simulink model "43_BusNetworkElectricityTransmissionModel"  (R2023b)
settings: Solver=VariableStepAuto  StartTime=0.0  StopTime=0.8  RelTol=1e-3
model workspace (MAT data in the model file):
  BESS_Fp_KDroop = 0.025
  BESS_KSI = 817
  BESS_PWM_fs = 560
  BESS_P_Ki = 0.5
  BESS_P_Kp = 0.0636
  BESS_Pnom = 3000000
  BESS_Q_Ki = 1
  BESS_Q_Kp = 0.0257
  BESS_Vd_Ki = 850
  BESS_Vd_Kp = 0.216
  BESS_Vnom = 1000
  BESS_Vq_KDroop = 0.025
  BESS_Vq_Ki = 850
  BESS_Vq_Kp = 0.216
  Compensation_Ki = 30
  Compensation_Kp = 3
  DC_Ki = 400
  DC_Kp = 8
  F = 0.01
  Flux_min = 0.5
  Grid_Freq_PWM = 2700
  Grid_Ireg_Ki = 5
  Grid_Ireg_Kp = 0.83
  Grid_Ireg_lim = 1.1
  Grid_Modindex_Upper = 1.1
  Grid_conv_Imax = 0.8
  H = 0.685
  Idref_max = 0.9
  Iqref_Tc = 0.3
  Ki_Var = 0.05
  Ki_Vreg = 20
  Ksh = 1.1
  L_pu = 0.3
  Llr = 0.16
  Lls = 0.18
  Lm = 2.9
  LowLoad_P = 130
  Nb_wt = 6
  P_mech = 1080000
  PeakShav_P = 200
  Pitch_Ki = 0
  Pitch_Kp = 150
  Pitch_Max = 27
  Pitch_Tc = 0.01
  Pitch_rate = 10
  Q_Filt = 50
  R_pu = 0.003
  Rotor_Freq_PWM = 1620
  Rotor_Ireg_Ki = 8
  Rotor_Ireg_Kp = 0.6
  Rotor_Ireg_lim = 0.1
  Rotor_Modindex_Upper = 2
  Rr = 0.016
  Rs = 0.023
  SOCBESS = Simulink.Parameter
  SOCBESS.DataType = 'auto'
  SOCBESS.Complexity = 'real'
  SOCBESS.Dimensions = [0 0]
  T_set = 0.0001
  Tp = 5e-05
  Ts = 5e-06
  Var_C_Filt = 720000
  Var_reg_max = 1.1
  Var_reg_min = 0.9
  WT_Coeff = [0.645 116 0.4 5 21 0.00912 0.08 0.035]
  WT_H = 4.32
  WT_IGBTRon = 5.931
  WT_Param = [91.204 10143]
  Wind_Freq_Filt = 10000
  Wind_Freq_nom = 60
  Wind_P_nom = 1200000
  Wind_Rotor_V_nom = 1950
  Wind_V_nom = 500
  Zeta_Filt = 0.707106781187
  init = [-0.2 0 0 0 0 0 0 0]
  p = 3
  torque0 = 0.83
  v_Ki = 0.1
  v_Kp = 3.6
  v_Max = 1.2
  v_Min = 0.7
  v_T = 5
  vreg_max = 1
  wind_VDC_nom = 1150
  wt0 = 1.2
undefined symbols (not defined in the file): D1, D11, Delta, DiscIntNeverNeededParam, Iabc, Ion, Lithium, P, Q, Vabc
libraries: powerlib_extras x156, spsSeriesRLCBranchLib x66, spsLoadFlowBusLib x43, spsThreePhaseSeriesRLCLoadLib x33, spsThreePhaseTransformerTwoWindingsLib x32, spsThreePhaseVIMeasurementLib x30, simulink_extras x30, spsDistributedParametersLineLib x22, spsGenericPowerSystemStabilizerLib x20, spsSynchronousMachinepuStandardLib x10, spsExcitationSystemLib x10, spsHydraulicTurbineandGovernorLib x10
(part 1 of 19)
settings Model: Creator=3.22  LastModifiedBy=3.22

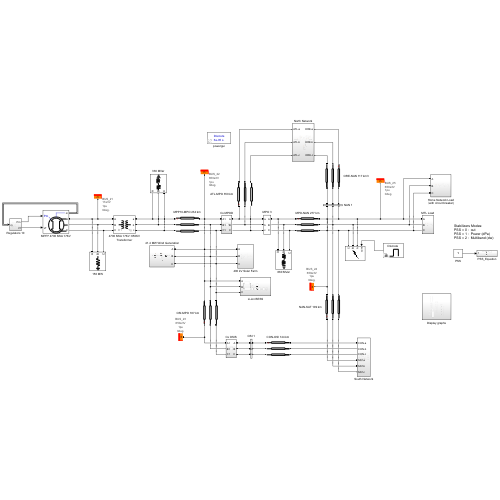
[thumbnail: Simulink's stored preview of the top-level diagram]
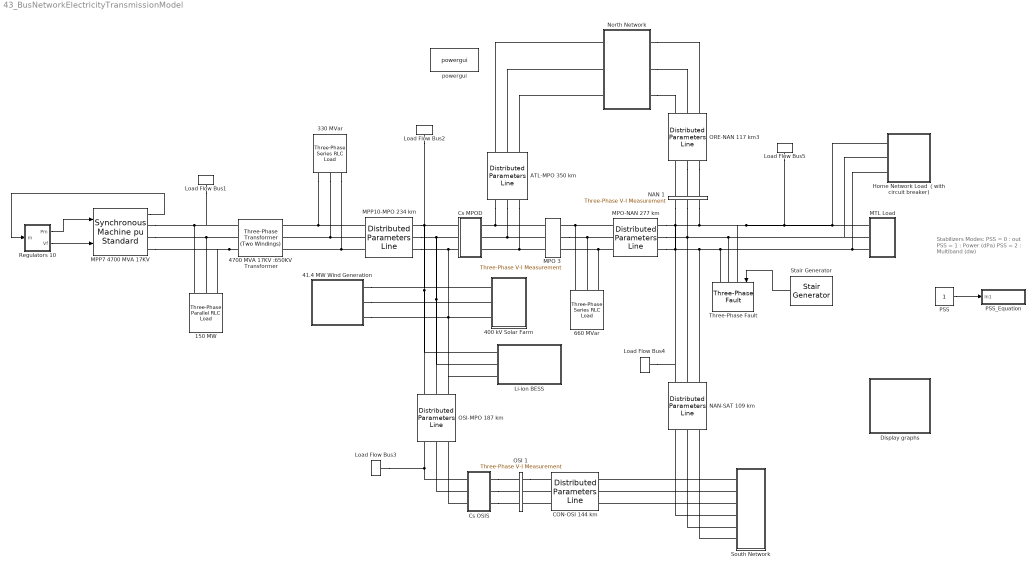
== system 43_BusNetworkElectricityTransmissionModel ==
  note: Stabilizers Modes:
      | PSS = 0 :  out
      | PSS = 1 :  Power (dPa)
      | PSS = 2 :  Multiband (dw)
  " 41.4 MW Wind Generation" : Subsystem
  150 MW : spsThreePhaseParallelRLCLoadLib/Three-Phase Parallel RLC Load  LConnTagsString=A|B|C  Configuration=Y (grounded)  NominalVoltage=17000  Vabc=[1e3 1e3 1e3]  Vabcp=[1e3 1e3 1e3]  NominalFrequency=60  UnbalancedPower=off  ActivePower=150e6  InductivePower=0  CapacitivePower=0  Pabc=[10e3 9e3 11e3]  QLabc=[100 90 110]  QCabc=[100 90 110]  Pabcp=[10e3 9e3 11e3]  QLabcp=[100 90 110]  QCabcp=[100 90 110]  Measurements=None  LoadType=constant Z
  330 MVar : spsThreePhaseSeriesRLCLoadLib/Three-Phase Series RLC Load  LConnTagsString=A|B|C  Configuration=Y (grounded)  NominalVoltage=650e3  Vabc=[1e3 1e3 1e3]  Vabcp=[1e3 1e3 1e3]  NominalFrequency=60  UnbalancedPower=off  ActivePower=1100e3  InductivePower=330e6  CapacitivePower=0  Pabc=[10e3 9e3 11e3]  QLabc=[100 90 110]  QCabc=[100 90 110]  Pabcp=[10e3 9e3 11e3]  QLabcp=[100 90 110]  QCabcp=[100 90 110]  Measurements=None  LoadType=constant Z
  400 kV Solar Farm : Subsystem
  "4700 MVA 17KV :650KV Transformer " : spsThreePhaseTransformerTwoWindingsLib/Three-Phase Transformer (Two Windings)  Winding1Connection=Delta (D1)  Winding2Connection=Yg  CoreType=Three single-phase transformers  SetSaturation=off  Hysteresis=off  DataFile='hysteresis'  SetInitialFlux=off  Measurements=None  UNITS=pu  NominalPower=[ 4700e6 , 60 ]  Winding1=[ 17e3 , 0.002 , 0.08 ]  Winding2=[ 650e3 , 0.002 , 0.08 ]  Rm=500  Lm=500  L0=0.5  Saturation=[ 0,0 ; 0.0024,1.2 ; 1.0,1.52 ]  InitialFluxes=[ 0.8 , -0.8 , 0.7 ]  BreakLoop=off  DiscreteSolver=Trapezoidal iterative  DataType=off  TransfoNumber=1
  660 MVar : spsThreePhaseSeriesRLCLoadLib/Three-Phase Series RLC Load  LConnTagsString=A|B|C  Configuration=Y (grounded)  NominalVoltage=650e3  Vabc=[1e3 1e3 1e3]  Vabcp=[1e3 1e3 1e3]  NominalFrequency=60  UnbalancedPower=off  ActivePower=2200e3  InductivePower=660e6  CapacitivePower=0  Pabc=[10e3 9e3 11e3]  QLabc=[100 90 110]  QCabc=[100 90 110]  Pabcp=[10e3 9e3 11e3]  QLabcp=[100 90 110]  QCabcp=[100 90 110]  Measurements=None  LoadType=constant Z
  ATL-MPO 350 km : spsDistributedParametersLineLib/Distributed Parameters Line  Phases=3  Length=350  Frequency=60  Resistance=[0.01273 0.3864]/6  Inductance="[0.9337e-3  4.1264e-3]/6"  Capacitance=[12.74e-9 7.751e-9]*6  x1=[-0.00198 6.71985344224008e-09 -287571.845218076 -158091.891979352;-0.00192 6.70807661913084e-09 -283922.60888035 -164555.645992495;-0.00186 6.69286782007226e-09 -280128.112489635 -170935.210296509;-0.0018 6.67423482616695e-09 -276190.297380398 -177227.320988416;-0.00174 6.65218717039889e-09 -272111.17821161 -183428.758908121;-0.00168 6.62673613275617e-09 -267892.841936014 -189536.351285395;-0.00162 6.59789473445993e-09 -263537.446732392 -195546.973363122;-0.00156 6.56567773130246e-09 -259047.22090141 -201457.549995984;-0.0015 6.53010160609788e-09 -254424.461725573 -207265.05722376;-0.00144 6.49118456024921e-09 -249671.534293893 -212966.523818443;-0.00138 6.44894650443622e-09 -244790.870291869 -218559.032804371;-0.00132 6.40340904842874e-09 -239784.966757388 -224039.722950611;-0.00126 6.35459549003068e-09 -234656.384803197 -229405.79023481;-0.0012 6.30253080316049e-09 -229407.74830659 -234654.489277794;-0.00114 6.24724162507404e-09 -224041.742566981 -239783.134748147;-0.00108 6.18875624273644e-09 -218561.11293206 -244789.102736079;-0.00102 6.12710457834999e-09 -212968.663393218 -249669.83209587;-0.00096 6.06231817404538e-09 -207267.255150975 -254422.825756192;-0.0009 5.99443017574417e-09 -201459.805151138 -259045.651997664;-0.00084 5.92347531620071e-09 -195549.284592437 -263535.94569696;-0.00078 5.84948989723225e-09 -189538.717406403 -267891.409536854;-0.00072 5.77251177114621e-09 -183431.178710271 -272109.815181565;-0.00066 5.69258032137431e-09 -177229.793233693 -276189.004416817;-0.0006 5.6097364423232e-09 -170937.733720066 -280126.890254024;-0.00054 5.52402251845218e-09 -164558.219303301 -283921.457998027;-0.00048 5.43548240258853e-09 -158094.513860855 -287570.766277852;-0.00042 5.34416139349154e-09 -151549.924343867 -291072.948039954;-0.00036 5.25010621267689e-09 -144927.799085264 -294426.211503428;-0.0003 5.15336498051303e-09 -138231.526086691 -297628.841076726;-0.00024 5.05398719160191e-09 -131464.531285147 -300679.198235381;-0.00018 4.95202368945661e-09 -124630.276800213 -303575.722360306;-0.00012 4.84752664048891e-09 -117732.259162765 -306316.931536237;-6e-05 4.74054950731994e-09 -110774.007526087 -308901.423309907]  x2=[-0.00198 2.79653655239106e-09 -267672.30015696 -181652.17479948;-0.00192 2.55125047403786e-09 -263495.280738514 -187659.824526183;-0.00186 2.30465912880045e-09 -259183.45226561 -193571.464019103;-0.0018 2.05688867736754e-09 -254739.020749366 -199384.068774241;-0.00174 1.80806588368036e-09 -250164.260043072 -205094.664955601;-0.00168 1.55831805007787e-09 -245461.510678835 -210700.330916655;-0.00162 1.30777295216655e-09 -240633.178670128 -216198.198695118;-0.00156 1.05655877344804e-09 -235681.734280824 -221585.455480246;-0.0015 8.04804039738072e-10 -230609.710761363 -226859.345051921;-0.00144 5.52637553410303e-10 -225419.7030527 -232017.169190789;-0.00138 3.00188327498644e-10 -220114.366458677 -237056.289058714;-0.00132 4.75855196917935e-11 -214696.415287529 -241974.126548861;-0.00126 -2.05041633746211e-10 -209168.621463186 -246768.165604697;-0.0012 -4.57563884095656e-10 -203533.81310711 -251435.953507259;-0.00114 -7.0985203630719e-10 -197794.873091376 -255975.102130004;-0.00108 -9.61777015100393e-10 -191954.73756374 -260383.289160623;-0.00102 -1.21320993100107e-09 -186016.394445451 -264658.259289177;-0.00096 -1.46402214628351e-09 -179982.881902575 -268797.825361957;-0.0009 -1.71408534078389e-09 -173857.286791617 -272799.869500469;-0.00084 -1.96327157755127e-09 -167642.743080223 -276662.344184983;-0.00078 -2.21145336830249e-09 -161342.430243787 -280383.273302079;-0.00072 -2.45850373864752e-09 -154959.571638773 -283960.753155667;-0.00066 -2.70429629305194e-09 -148497.432853586 -287392.953440949;-0.0006 -2.94870527950318e-09 -141959.320037833 -290678.118180839;-0.00054 -3.19160565384762e-09 -135348.578210842 -293814.566624354;-0.00048 -3.43287314376546e-09 -128668.589550285 -296800.694106514;-0.00042 -3.67238431235074e-09 -121922.771661791 -299634.972869324;-0.00036 -3.91001662126397e-09 -115114.575830441 -302315.952843396;-0.0003 -4.14564849342495e-09 -108247.485255024 -304842.262389837;-0.00024 -4.37915937521393e-09 -101325.013265967 -307212.609002002;-0.00018 -4.61042979814898e-09 -94350.7015278514 -309425.779966765;-0.00012 -4.83934144000835e-09 -87328.118227434 -311480.642984966;-6e-05 -5.06577718536627e-09 -80260.8562480934 -313376.146750715]  x3=[-0.00198 1.49045766658214e-10 -8241.07227031755 -3031.05749753974;-0.00192 1.47930956165664e-10 -8170.40834869366 -3216.6754938586;-0.00186 1.46740461462489e-10 -8095.56429518679 -3400.64777955748;-0.0018 1.45474891627779e-10 -8016.57840139768 -3582.88023101559;-0.00174 1.44134894150444e-10 -7933.49107796907 -3763.27961474349;-0.00168 1.42721154597956e-10 -7846.34483391092 -3941.75363508309;-0.00162 1.41234396265592e-10 -7755.18425485195 -4118.21098142774;-0.00156 1.39675379806387e-10 -7660.05598022887 -4292.5613749385;-0.0015 1.38044902841968e-10 -7561.00867942474 -4464.71561473243;-0.00144 1.36343799554479e-10 -7458.09302686885 -4634.5856235194;-0.00138 1.34572940259794e-10 -7351.36167611069 -4802.08449266409;-0.00132 1.3273323096225e-10 -7240.86923288149 -4967.12652665;-0.00126 1.30825612891118e-10 -7126.67222715687 -5129.62728692295;-0.0012 1.28851062019051e-10 -7008.82908423508 -5289.50363509128;-0.00114 1.26810588562762e-10 -6887.40009484551 -5446.67377546111;-0.00108 1.24705236466173e-10 -6762.44738430291 -5601.05729688446;-0.00102 1.22536082866321e-10 -6634.03488072283 -5752.57521389908;-0.00096 1.20304237542268e-10 -6502.22828231491 -5901.15000713891;-0.0009 1.18010842347321e-10 -6367.09502377039 -6046.70566299436;-0.00084 1.1565707062484e-10 -6228.70424176131 -6189.16771250235;-0.00078 1.1324412660793e-10 -6087.12673956894 -6328.46326944596;-0.00072 1.10773244803337e-10 -5942.43495085943 -6464.52106764436;-0.00066 1.08245689359848e-10 -5794.70290262548 -6597.27149741394;-0.0006 1.05662753421532e-10 -5644.00617731276 -6726.64664118189;-0.00054 1.03025758466143e-10 -5490.42187415047 -6852.58030823406;-0.00048 1.00336053629025e-10 -5334.02856970605 -6975.00806857942;-0.00042 9.75950150128734e-11 -5174.90627768384 -7093.86728591356;-0.00036 9.48040449836927e-11 -5013.1364079887 -7209.09714966463;-0.0003 9.19645714533211e-11 -4848.80172507512 -7320.63870610513;-0.00024 8.9078047148884e-11 -4681.98630560344 -7428.43488851374;-0.00018 8.61459488695525e-11 -4512.77549542465 -7532.4305463717;-0.00012 8.31697767309852e-11 -4341.25586591589 -7632.57247357881;-6e-05 8.01510533978416e-11 -4167.51516968895 -7728.80943567472]  x4=[-0.00198 -4.77653400589125e-11 -5640.6008243666 -1578.68999483631;-0.00192 -4.78138362701717e-11 -5603.45127275738 -1705.86309036725;-0.00186 -4.78378700392969e-11 -5563.43489193714 -1832.16343482044;-0.0018 -4.78374290701678e-11 -5520.57215502573 -1957.52641060589;-0.00174 -4.78125135883924e-11 -5474.88499139136 -2081.88787970874;-0.00168 -4.77631363411914e-11 -5426.39677543116 -2205.18421650347;-0.00162 -4.76893225908771e-11 -5375.13231461236 -2327.35234030591;-0.00156 -4.75911101019278e-11 -5321.11783678037 -2448.32974764653;-0.0015 -4.74685491216678e-11 -5264.38097674014 -2568.05454424832;-0.00144 -4.73217023545593e-11 -5204.95076211764 -2686.46547669308;-0.00138 -4.71506449301216e-11 -5142.8575985088 -2803.50196375979;-0.00132 -4.69554643644939e-11 -5078.13325392348 -2919.10412741908;-0.00126 -4.67362605156601e-11 -5010.81084253234 -3033.21282346794;-0.0012 -4.64931455323597e-11 -4940.92480772502 -3145.76967178898;-0.00114 -4.62262437967104e-11 -4868.51090448828 -3256.7170862188;-0.00108 -4.59356918605719e-11 -4793.60618111307 -3365.9983040101;-0.00102 -4.56216383756836e-11 -4716.24896023993 -3473.55741487256;-0.00096 -4.52842440176113e-11 -4636.47881925248 -3579.33938957762;-0.0009 -4.4923681403543e-11 -4554.33657002882 -3683.29010811238;-0.00084 -4.45401350039744e-11 -4469.86423806147 -3785.35638736845;-0.00078 -4.41338010483308e-11 -4383.10504095633 -3885.4860083514;-0.00072 -4.37048874245719e-11 -4294.10336632177 -3983.62774289696;-0.00066 -4.32536135728331e-11 -4202.9047490591 -4079.73137988027;-0.0006 -4.27802103731556e-11 -4109.55584806605 -4173.74775090486;-0.00054 -4.22849200273638e-11 -4014.10442236527 -4265.6287554581;-0.00048 -4.17679959351505e-11 -3916.59930666989 -4355.3273855203;-0.00042 -4.1229702564433e-11 -3817.09038639878 -4442.79774961486;-0.00036 -4.06703153160462e-11 -3715.62857215427 -4527.99509628725;-0.0003 -4.00901203828427e-11 -3612.26577367532 -4610.87583700066;-0.00024 -3.9489414603271e-11 -3507.05487327957 -4691.39756843667;-0.00018 -3.88685053095079e-11 -3400.04969880772 -4769.5190941896;-0.00012 -3.8227710170221e-11 -3291.30499608426 -4845.20044584337;-6e-05 -3.75673570280441e-11 -3180.87640090849 -4918.40290342003]  x5=0.0019793954844851  V1=[4.219e-16 0.0001256 0.0001256;377 377 377;2.896 1.02 -0.5506]  V2=[3.447e-16 8.016e-05 8.016e-05;377 377 377;2.788 1.015 -0.5555]  I1=[4.128e-19 5.188e-07 5.188e-07;377 377 377;2.697 1.572 0.0007381]  I2=[5.884e-19 5.436e-07 5.436e-07;377 377 377;2.289 0.05248 -1.518]  nHarmo=1  Measurements=None  Decoupling=off  VsMag0=0  VrMag0=0  VsAngle0=0  VrAngle0=0  IsMag0=0  IrMag0=0  IsAngle0=0  IrAngle0=0
      settings: LibrarySourceBlock=sps_lib/Power Grid Elements/Distributed Parameters Line
  CON-OSI 144 km : spsDistributedParametersLineLib/Distributed Parameters Line  Phases=3  Length=144  Frequency=60  Resistance=[0.01273 0.3864]/6  Inductance="[0.9337e-3  4.1264e-3]/6"  Capacitance=[12.74e-9 7.751e-9]*6  x1=[-0.00084 1.11335894760226e-08 0 0;-0.00078 1.11391421976134e-08 0 0;-0.00072 1.11389959282283e-08 0 0;-0.00066 1.11331507427013e-08 0 0;-0.0006 1.11216096315373e-08 0 0;-0.00054 1.11043784993822e-08 -161806.103434456 -299072.25041941;-0.00048 1.10814661620014e-08 -155000.429702794 -302655.438182157;-0.00042 1.10528843417702e-08 -148115.454887217 -306083.7818303;-0.00036 1.10186476616759e-08 -141154.701468061 -309355.527359881;-0.0003 1.09787736378367e-08 -134121.730695395 -312469.000885432;-0.00024 1.093328267054e-08 -127020.14076702 -315422.609496367;-0.00018 1.08821980338052e-08 -119853.564987567 -318214.842071943;-0.00012 1.08255458634764e-08 -112625.669909627 -320844.270054381;-6e-05 1.07633551438508e-08 -105340.153457878 -323309.548179739]  x2=[-0.00084 1.46810325444429e-08 0 0;-0.00078 1.47653085837444e-08 0 0;-0.00072 1.4842030418343e-08 0 0;-0.00066 1.49111587959304e-08 0 0;-0.0006 1.49726583491513e-08 0 0;-0.00054 1.50264976136978e-08 -156401.510226705 -298797.35932392;-0.00048 1.50726490444074e-08 -149603.436972216 -302258.378507116;-0.00042 1.51110890293553e-08 -142728.823835017 -305564.756718775;-0.00036 1.5141797901935e-08 -135781.187994219 -308714.802354709;-0.0003 1.51647599509198e-08 -128764.083988696 -311706.903793365;-0.00024 1.51799634285012e-08 -121681.101898517 -314539.530220358;-0.00018 1.51874005562991e-08 -114535.865508198 -317211.232411669;-0.00012 1.51870675293414e-08 -107332.030452706 -319720.643475088;-6e-05 1.51789645180111e-08 -100073.282347167 -322066.479549548]  x3=[-0.00084 1.97530423019833e-11 0 0;-0.00078 2.26448699855483e-11 0 0;-0.00072 2.55251121351995e-11 0 0;-0.00066 2.83922951658325e-11 0 0;-0.0006 3.12449521736294e-11 0 0;-0.00054 3.40816236865539e-11 -4132.59337571189 -6898.49195009985;-0.00048 3.69008584110444e-11 -3975.50918349761 -6990.1972251609;-0.00042 3.97012139745224e-11 -3816.39104732609 -7078.32618615756;-0.00036 4.24812576633368e-11 -3655.32037497595 -7162.83374468495;-0.0003 4.52395671557674e-11 -3492.37957317942 -7243.67666511461;-0.00024 4.79747312497099e-11 -3327.6520054615 -7320.81358671464;-0.00018 5.0685350584674e-11 -3161.22194948965 -7394.20504481063;-0.00012 5.33700383577214e-11 -2993.17455395577 -7463.81349097649;-6e-05 5.602742103298e-11 -2823.59579501258 -7529.60331224495]  x4=[-0.00084 1.76672604781152e-10 0 0;-0.00078 1.752749503463e-10 0 0;-0.00072 1.73787622008142e-10 0 0;-0.00066 1.72211380711339e-10 0 0;-0.0006 1.70547032890063e-10 0 0;-0.00054 1.68795430055414e-10 -4123.99782512585 -5624.97159291165;-0.00048 1.66957468359768e-10 -3995.71966323754 -5716.80809743081;-0.00042 1.65034088138289e-10 -3865.39721733711 -5805.71977729286;-0.00036 1.6302627342784e-10 -3733.09716279596 -5891.66114363949;-0.0003 1.60935051463526e-10 -3598.88718676662 -5974.58822727964;-0.00024 1.58761492153145e-10 -3462.83595355274 -6054.45860118503;-0.00018 1.56506707529804e-10 -3325.01306947917 -6131.23140219651;-0.00012 1.54171851182979e-10 -3185.48904728008 -6204.8673519305;-6e-05 1.5175811766832e-10 -3044.33527002333 -6275.32877687447]  x5=0.000814379856473869  V1=[3.066e-13 0.3294 0.3294;377 377 377;-0.5534 -1.851 2.861]  V2=[2.167e-13 0.2213 0.2213;377 377 377;-0.5727 -1.852 2.86]  I1=[4.19e-16 0.002316 0.002316;377 377 377;0.2564 -0.79 -2.361]  I2=[5.677e-16 0.002387 0.002387;377 377 377;-1.374 -3.038 1.674]  nHarmo=1  Measurements=None  Decoupling=off  VsMag0=0  VrMag0=0  VsAngle0=0  VrAngle0=0  IsMag0=0  IrMag0=0  IsAngle0=0  IrAngle0=0
      settings: LibrarySourceBlock=sps_lib/Power Grid Elements/Distributed Parameters Line
  Cs MPOD : Subsystem
  Cs OSIS : Subsystem
  Display graphs : Subsystem
  Home Network Load （with circuit breaker) : Subsystem
  Li-ion BESS : Subsystem
  Load Flow Bus1 : spsLoadFlowBusLib/Load Flow Bus  LConnTagsString=a  Phases=single  Connectors=on one side  ID=BUS_21  Vbase=17e3  Vref=1  Vangle=0  VLF=1  VLFb=1  VLFc=1  angleLF=0  angleLFb=0  angleLFc=0
  Load Flow Bus2 : spsLoadFlowBusLib/Load Flow Bus  LConnTagsString=a  Phases=single  Connectors=on one side  ID=BUS_22  Vbase=650e3  Vref=1  Vangle=0  VLF=1  VLFb=1  VLFc=1  angleLF=0  angleLFb=0  angleLFc=0
  Load Flow Bus3 : spsLoadFlowBusLib/Load Flow Bus  LConnTagsString=a  Phases=single  Connectors=on one side  ID=BUS_23  Vbase=650e3  Vref=1  Vangle=0  VLF=1  VLFb=1  VLFc=1  angleLF=0  angleLFb=0  angleLFc=0
  Load Flow Bus4 : spsLoadFlowBusLib/Load Flow Bus  LConnTagsString=a  Phases=single  Connectors=on one side  ID=BUS_24  Vbase=650e3  Vref=1  Vangle=0  VLF=1  VLFb=1  VLFc=1  angleLF=0  angleLFb=0  angleLFc=0
  Load Flow Bus5 : spsLoadFlowBusLib/Load Flow Bus  LConnTagsString=a  Phases=single  Connectors=on one side  ID=BUS_25  Vbase=650e3  Vref=1  Vangle=0  VLF=1  VLFb=1  VLFc=1  angleLF=0  angleLFb=0  angleLFc=0
  MPO 3 : spsThreePhaseVIMeasurementLib/Three-Phase V-I Measurement  VoltageMeasurement=no  SetLabelV=off  LabelV=Vabc_MPO3  Vpu=off  VpuLL=off  CurrentMeasurement=no  SetLabelI=off  LabelI=Iabc  Ipu=off  Pbase=100e6  Vbase=500e3  OutputType=Complex  PhasorSimulation=off  PSBequivalent=0
  MPO-NAN 277 km : spsDistributedParametersLineLib/Distributed Parameters Line  Phases=3  Length=277  Frequency=60  Resistance=[0.01273 0.3864]/6  Inductance="[0.9337e-3  4.1264e-3]/6"  Capacitance=[12.74e-9 7.751e-9]*6  x1=[-0.00162 6.59789473445993e-09 -263537.446732392 -195546.973363122;-0.00156 6.56567773130246e-09 -259047.22090141 -201457.549995984;-0.0015 6.53010160609788e-09 -254424.461725573 -207265.05722376;-0.00144 6.49118456024921e-09 -249671.534293893 -212966.523818443;-0.00138 6.44894650443622e-09 -244790.870291869 -218559.032804371;-0.00132 6.40340904842874e-09 -239784.966757388 -224039.722950611;-0.00126 6.35459549003068e-09 -234656.384803197 -229405.79023481;-0.0012 6.30253080316049e-09 -229407.74830659 -234654.489277794;-0.00114 6.24724162507404e-09 -224041.742566982 -239783.134748147;-0.00108 6.18875624273644e-09 -218561.11293206 -244789.102736079;-0.00102 6.12710457834999e-09 -212968.663393218 -249669.83209587;-0.00096 6.06231817404538e-09 -207267.255150975 -254422.825756192;-0.0009 5.99443017574417e-09 -201459.805151138 -259045.651997664;-0.00084 5.92347531620071e-09 -195549.284592437 -263535.94569696;-0.00078 5.84948989723225e-09 -189538.717406403 -267891.409536854;-0.00072 5.77251177114621e-09 -183431.178710271 -272109.815181565;-0.00066 5.69258032137431e-09 -177229.793233693 -276189.004416817;-0.0006 5.6097364423232e-09 -170937.733720066 -280126.890254024;-0.00054 5.52402251845218e-09 -164558.219303301 -283921.457998027;-0.00048 5.43548240258853e-09 -158094.513860855 -287570.766277852;-0.00042 5.34416139349154e-09 -151549.924343867 -291072.948039954;-0.00036 5.25010621267689e-09 -144927.799085264 -294426.211503428;-0.0003 5.15336498051303e-09 -138231.526086691 -297628.841076726;-0.00024 5.05398719160191e-09 -131464.531285147 -300679.198235381;-0.00018 4.95202368945661e-09 -124630.276800213 -303575.722360306;-0.00012 4.84752664048891e-09 -117732.259162765 -306316.931536237;-6e-05 4.74054950731994e-09 -110774.007526087 -308901.423309907]  x2=[-0.00162 1.65325802312698e-08 -236183.487157273 -173158.041325444;-0.00156 1.60010574522097e-08 -232206.645197303 -178455.662809894;-0.0015 1.54613482364915e-08 -228111.002026965 -183661.983079769;-0.00144 1.49137287093227e-08 -223898.653052983 -188774.338485417;-0.00138 1.43584790429721e-08 -219571.753390928 -193790.113451348;-0.00132 1.3795883313429e-08 -215132.516762618 -198706.741814407;-0.00126 1.32262293550641e-08 -210583.214363541 -203521.708136676;-0.0012 1.26498086133685e-08 -205926.173700865 -208232.548992413;-0.00114 1.20669159958447e-08 -201163.777402645 -212836.85422839;-0.00108 1.14778497211265e-08 -196298.461998827 -217332.268196971;-0.00102 1.08829111664047e-08 -191332.716674672 -221716.490961304;-0.00096 1.02824047132371e-08 -186269.081997244 -225987.279472012;-0.0009 9.6766375918212e-09 -181110.148615609 -230142.448714777;-0.00084 9.06591972380962e-09 -175858.555935412 -234179.872828236;-0.00078 8.45056356374839e-09 -170516.990768506 -238097.486191609;-0.00072 7.8308839392195e-09 -165088.185958331 -241893.284481511;-0.00066 7.2071978897692e-09 -159574.91898174 -245565.325697399;-0.0006 6.57982450470479e-09 -153980.010527993 -249111.731155134;-0.00054 5.94908475984259e-09 -148306.323055637 -252530.686448154;-0.00048 5.31530135329082e-09 -142556.759328019 -255820.442375758;-0.00042 4.67879854035122e-09 -136734.260928183 -258979.315838023;-0.00036 4.03990196762412e-09 -130841.806753898 -262005.690696918;-0.0003 3.39893850640158e-09 -124882.411493599 -264898.018603144;-0.00024 2.756236085434e-09 -118859.124084018 -267654.8197883;-0.00018 2.11212352315573e-09 -112775.026150291 -270274.68382196;-0.00012 1.46693035945546e-09 -106633.230429344 -272756.270333275;-6e-05 8.20986687077529e-10 -100436.879177353 -275098.309696731]  x3=[-0.00162 3.6702576124587e-10 -5110.22111110319 -4892.66765470672;-0.00156 3.68472786391517e-10 -4998.25343123766 -5006.99753010207;-0.0015 3.69731294051052e-10 -4883.72855255961 -5118.76573304235;-0.00144 3.70800640348701e-10 -4766.70506811315 -5227.9150808497;-0.00138 3.7168027818714e-10 -4647.24284927525 -5334.38973070091;-0.00132 3.72369757527397e-10 -4525.40301512449 -5438.13520819771;-0.00126 3.72868725619101e-10 -4401.24790117136 -5539.09843523681;-0.0012 3.73176927180956e-10 -4274.84102746628 -5637.22775716567;-0.00114 3.73294204531348e-10 -4146.24706610157 -5732.47296920997;-0.00108 3.73220497669019e-10 -4015.531808124 -5824.78534215931;-0.00102 3.7295584430376e-10 -3882.7621298749 -5914.11764729794;-0.00096 3.72500379837124e-10 -3748.00595877497 -6000.42418056787;-0.0009 3.71854337293147e-10 -3611.33223857133 -6083.66078595195;-0.00084 3.71018047199133e-10 -3472.8108940647 -6163.7848780648;-0.00078 3.69991937416547e-10 -3332.51279533449 -6240.75546394038;-0.00072 3.68776532922113e-10 -3190.50972148043 -6314.53316400471;-0.00066 3.6737245553923e-10 -3046.87432389903 -6385.08023222318;-0.0006 3.6578042361983e-10 -2901.68008911375 -6452.36057541212;-0.00054 3.64001251676861e-10 -2755.001301178 -6516.33977170477;-0.00048 3.62035849967565e-10 -2606.91300366999 -6576.9850881621;-0.00042 3.59885224027772e-10 -2457.4909612991 -6634.26549751962;-0.00036 3.57550474157452e-10 -2306.81162114319 -6688.15169406147;-0.0003 3.5503279485778e-10 -2154.95207353692 -6738.6161086138;-0.00024 3.52333474220006e-10 -2001.9900126309 -6785.63292264966;-0.00018 3.49453893266448e-10 -1848.0036966419 -6829.17808149822;-0.00012 3.46395525243929e-10 -1693.07190781451 -6869.22930665157;-6e-05 3.43159934870042e-10 -1537.27391211471 -6905.76610716288]  x4=[-0.00162 -1.35947067479577e-10 -7334.42415124215 -1195.49642544369;-0.00156 -1.40386272478209e-10 -7305.50809254828 -1361.07753565119;-0.0015 -1.44753653265802e-10 -7272.854400924 -1525.96229344163;-0.00144 -1.49046975409643e-10 -7236.4797826013 -1690.06634072621;-0.00138 -1.53264042366794e-10 -7196.40284750705 -1853.30571884203;-0.00132 -1.57402696607876e-10 -7152.64409974178 -2015.59691150694;-0.00126 -1.61460820720905e-10 -7105.22592708941 -2176.85688754798;-0.0012 -1.65436338494601e-10 -7054.17258956327 -2337.00314338166;-0.00114 -1.69327215980611e-10 -6999.51020699418 -2495.95374522433;-0.00108 -1.73131462534119e-10 -6941.26674566712 -2653.62737101102;-0.00102 -1.76847131832292e-10 -6879.47200401311 -2809.9433520013;-0.00096 -1.8047232287006e-10 -6814.15759736383 -2964.82171405092;-0.0009 -1.84005180932703e-10 -6745.35694177657 -3118.18321852802;-0.00084 -1.87443898544757e-10 -6673.10523693804 -3269.94940285312;-0.00078 -1.90786716394749e-10 -6597.43944815548 -3420.04262064201;-0.00072 -1.94031924235301e-10 -6518.39828744458 -3568.38608143105;-0.00066 -1.97177861758116e-10 -6436.02219372367 -3714.90388996464;-0.0006 -2.00222919443428e-10 -6350.35331212444 -3859.52108502459;-0.00054 -2.03165539383459e-10 -6261.43547242968 -4002.1636777817;-0.00048 -2.06004216079473e-10 -6169.31416664921 -4142.75868964977;-0.00042 -2.08737497212021e-10 -6074.03652574526 -4281.23418962283;-0.00036 -2.11363984383969e-10 -5975.65129551945 -4417.51933107637;-0.0003 -2.1388233383595e-10 -5874.20881167351 -4551.54438801376;-0.00024 -2.16291257133849e-10 -5769.76097405662 -4683.24079073938;-0.00018 -2.18589521827995e-10 -5662.36122011247 -4812.5411609401;-0.00012 -2.20775952083704e-10 -5552.06449753971 -4939.37934615736;-6e-05 -2.22849429282857e-10 -5438.92723617966 -5063.69045363189]  x5=0.00156655014057821  V1=[4.219e-16 0.0001256 0.0001256;377 377 377;3.052 1.115 -0.4557]  V2=[4.095e-15 0.006804 0.006804;377 377 377;-1.109 1.061 -0.5096]  I1=[9.849e-18 6.958e-05 6.958e-05;377 377 377;-2.423 -0.4689 -2.04]  I2=[7.867e-18 6.871e-05 6.871e-05;377 377 377;0.191 2.298 0.7273]  nHarmo=1  Measurements=None  Decoupling=off  VsMag0=0  VrMag0=0  VsAngle0=0  VrAngle0=0  IsMag0=0  IrMag0=0  IsAngle0=0  IrAngle0=0
      settings: LibrarySourceBlock=sps_lib/Power Grid Elements/Distributed Parameters Line
  MPP10-MPO 234 km : spsDistributedParametersLineLib/Distributed Parameters Line  Phases=3  Length=234  Frequency=60  Resistance=[0.01273 0.3864]/6  Inductance="[0.9337e-3  4.1264e-3]/6"  Capacitance=[12.74e-9 7.751e-9]*6  x1=[-0.00138 4.2065148299145e-08 -199933.902069884 -213017.780521915;-0.00132 4.20168168193009e-08 -195064.806534314 -217485.331564361;-0.00126 4.19469887595904e-08 -190095.912239338 -221841.613092511;-0.0012 4.18556998453393e-08 -185029.761363091 -226084.396352242;-0.00114 4.17429967816429e-08 -179868.945841974 -230211.510657239;-0.00108 4.16089372294711e-08 -174616.106044569 -234220.844499565;-0.00102 4.1453589776168e-08 -169273.929420776 -238110.346629941;-0.00096 4.12770339003611e-08 -163845.149126869 -241878.027107207;-0.0009 4.10793599312989e-08 -158332.542627159 -245521.958316414;-0.00084 4.08606690026365e-08 -152738.930272992 -249040.275955022;-0.00078 4.06210730006941e-08 -147067.173859805 -252431.179986716;-0.00072 4.03606945072133e-08 -141320.175162984 -255692.935562337;-0.00066 4.00796667366428e-08 -135500.874453252 -258823.873907462;-0.0006 3.97781334679827e-08 -129612.248992382 -261822.393176181;-0.00054 3.94562489712251e-08 -123657.311509968 -264686.959270629;-0.00048 3.9114177928426e-08 -117639.108662062 -267416.106625861;-0.00042 3.87520953494519e-08 -111560.719472443 -270008.438959663;-0.00036 3.83701864824406e-08 -105425.253757337 -272462.62998691;-0.0003 3.79686467190254e-08 -99235.8505343737 -274777.424098125;-0.00024 3.75476814943688e-08 -92995.6764166096 -276951.637001869;-0.00018 3.71075061820583e-08 -86707.9239924282 -278984.156330645;-0.00012 3.66483459839171e-08 -80375.8101921541 -280873.942210007;-6e-05 3.61704358147871e-08 -74002.5746422114 -282620.027790582]  x2=[-0.00138 6.30686550171584e-09 -239778.021913043 -223551.966975834;-0.00132 6.22310933391275e-09 -234660.47396165 -228918.001898516;-0.00126 6.1361693083846e-09 -229422.869375751 -234166.918141507;-0.0012 6.0460899052549e-09 -224067.887810633 -239296.030262271;-0.00114 5.95291721081078e-09 -218598.268973811 -244302.71411227;-0.00108 5.85669889392434e-09 -213016.811223352 -249184.408179534;-0.00102 5.75748418166442e-09 -207326.370136172 -253938.614899175;-0.00096 5.65532383411108e-09 -201529.85704708 -258562.901931187;-0.0009 5.55027011838585e-09 -195630.237559278 -263054.903404879;-0.00084 5.44237678191084e-09 -189630.530027111 -267412.321129292;-0.00078 5.33169902491065e-09 -183533.804011812 -271632.925769005;-0.00072 5.21829347217085e-09 -177343.178711066 -275714.557984694;-0.00066 5.1022181440677e-09 -171061.821363166 -279655.1295379;-0.0006 4.9835324268839e-09 -164692.945626598 -283452.624359401;-0.00054 4.86229704242542e-09 -158239.809935871 -287105.099580677;-0.00048 4.73857401695511e-09 -151705.715834446 -290610.686527916;-0.00042 4.61242664945895e-09 -145094.0062856 -293967.591678059;-0.00036 4.48391947926107e-09 -138408.06396211 -297174.097576403;-0.0003 4.3531182530043e-09 -131651.30951561 -300228.563715281;-0.00024 4.22008989101292e-09 -124827.199826525 -303129.427373376;-0.00018 4.084902453055e-09 -117939.226235468 -305875.204415239;-0.00012 3.94762510352178e-09 -110990.912757002 -308464.490050599;-6e-05 3.80832807604187e-09 -103985.814276693 -310895.959553081]  x3=[-0.00138 2.22134509345444e-10 -5992.2185827041 -1106.11035406549;-0.00132 2.11129797178613e-10 -5965.66763508576 -1241.35707554806;-0.00126 2.00017067106315e-10 -5936.06454167244 -1375.96869581314;-0.0012 1.88802004606596e-10 -5903.42444795375 -1509.87634506847;-0.00114 1.77490347512659e-10 -5867.76405320474 -1643.01151368635;-0.00108 1.66087883077291e-10 -5829.1016019423 -1775.30608725446;-0.00102 1.54600445011989e-10 -5787.45687459089 -1906.69238142446;-0.00096 1.43033910502332e-10 -5742.85117736253 -2037.10317654049;-0.0009 1.31394197201098e-10 -5695.30733135614 -2166.47175203006;-0.00084 1.19687260200691e-10 -5644.84966088186 -2294.7319205395;-0.00078 1.07919088986399e-10 -5591.50398101623 -2421.81806179662;-0.00072 9.60957043720655e-11 -5535.29758439481 -2547.66515618327;-0.00066 8.42231554197312e-11 -5476.25922724867 -2672.20881800058;-0.0006 7.23075163448192e-11 -5414.41911469223 -2795.38532840986;-0.00054 6.03548834084559e-11 -5349.80888526975 -2917.13166803235;-0.00048 4.83713717985108e-11 -5282.46159476847 -3037.38554919107;-0.00042 3.63631125009534e-11 -5212.41169930664 -3156.08544777839;-0.00036 2.43362491631274e-11 -5139.69503770515 -3273.17063473288;-0.0003 1.22969349505474e-11 -5064.34881315172 -3388.5812071094;-0.00024 2.51329398825468e-13 -4986.41157416707 -3502.25811872658;-0.00018 -1.17944047376609e-11 -4905.92319488279 -3614.14321037593;-0.00012 -2.3834104638748e-11 -4822.92485464098 -3724.17923957716;-6e-05 -3.58616105714983e-11 -4737.45901692612 -3832.30990986451]  x4=[-0.00138 1.5214404178847e-10 -5147.78715577902 -7003.66777552525;-0.00132 1.64242811244797e-10 -4988.06433756092 -7118.30729971566;-0.00126 1.76257551044034e-10 -4825.78953345889 -7229.30496636033;-0.0012 1.88182114223292e-10 -4661.0457662612 -7336.60398700202;-0.00114 2.00010399955707e-10 -4493.91732192327 -7440.1494654791;-0.00108 2.11736356671737e-10 -4324.4897064454 -7539.8884260115;-0.00102 2.23353985155257e-10 -4152.84960212633 -7635.76984030402;-0.00096 2.34857341612863e-10 -3979.08482321497 -7727.74465365344;-0.0009 2.46240540714836e-10 -3803.28427098302 -7815.76581004575;-0.00084 2.57497758606177e-10 -3625.53788824143 -7899.78827623089;-0.00078 2.68623235886204e-10 -3445.93661332397 -7979.7690647626;-0.00072 2.79611280555165e-10 -3264.57233356155 -8055.66725599161;-0.00066 2.90456270926371e-10 -3081.53783827092 -8127.44401900083;-0.0006 3.01152658502356e-10 -2896.92677128196 -8195.06263147204;-0.00054 3.1169497081359e-10 -2710.83358302775 -8258.48849847363;-0.00048 3.22077814218296e-10 -2523.35348222203 -8317.68917016009;-0.00042 3.32295876661933e-10 -2334.58238714858 -8372.63435837386;-0.00036 3.42343930394948e-10 -2144.61687658775 -8423.2959521414;-0.0003 3.52216834647385e-10 -1953.5541404049 -8469.64803205521;-0.00024 3.61909538258997e-10 -1761.49192982628 -8511.66688353472;-0.00018 3.71417082263517e-10 -1568.52850742774 -8549.33100895909;-0.00012 3.80734602425752e-10 -1374.76259686172 -8582.6211386658;-6e-05 3.8985733173022e-10 -1180.29333234845 -8611.52024080937]  x5=0.00132336726677004  V1=[5.094e-16 1.649e-05 1.649e-05;377 377 377;1.389 -1.935 2.777]  V2=[3.793e-13 0.4417 0.4417;377 377 377;-0.7025 -1.967 2.745]  I1=[9.917e-16 0.005412 0.005412;377 377 377;-2.043 2.781 1.21]  I2=[8.773e-16 0.005353 0.005353;377 377 377;0.5828 -0.6661 -2.237]  nHarmo=1  Measurements=None  Decoupling=off  VsMag0=0  VrMag0=0  VsAngle0=0  VrAngle0=0  IsMag0=0  IrMag0=0  IsAngle0=0  IrAngle0=0
      settings: LibrarySourceBlock=sps_lib/Power Grid Elements/Distributed Parameters Line
  MPP7 4700 MVA 17KV : spsSynchronousMachinepuStandardLib/Synchronous Machine pu Standard  PresetModel=No  MechanicalLoad=Mechanical power Pm  ShowDetailedParameters=on  RotorType=Salient-pole  Units=per unit standard parameters  MeasurementBus=off  NominalParameters=[2700e6 17000 60]  Reactances1=[ 1.81, 0.3, 0.23, 1.76, 0.65, 0.25, 0.15 ]  Reactances2=[ 1.305, 0.296, 0.252, 0.474, 0.243, 0.18 ]  dAxisTimeConstants=Short-circuit  qAxisTimeConstants=Open-circuit  TimeConstants1="[ 4.4849  0.0681  0.1  ]"  TimeConstants2=[ 8.0, 0.03, 1.0, 0.07 ]  TimeConstants3="[  4.49  0.0681  0.0513  ]"  TimeConstants4=[ 8.0, 0.03, 0.3371, 0.0295 ]  TimeConstants5=[ 1.01, 0.053, 0.1 ]  TimeConstants6=[ 1.3201, 0.023, 1.0, 0.07 ]  TimeConstants7=[0.012 0.003 0.003]  TimeConstants8=[ 1.3201, 0.0231, 0.3371, 0.0295 ]  StatorResistance=2.8544e-3  Mechanical=[3.5 0 32]  PolePairs=20  InitialConditions=[0 -81.9543 0.907703 0.907703 0.907703 -8.76021 -128.76 111.24 1.25655]  SetSaturation=off  Saturation=[0.6404,0.7127,0.8441,0.9214,0.9956,1.082,1.19,1.316,1.457;0.7,0.7698,0.8872,0.9466,0.9969,1.046,1.1,1.151,1.201]  LoadFlowParameters=[1,0,0,0,0]  TsPowergui=0  TsBlock=-1  IterativeModel=Trapezoidal non iterative  IterativeDiscreteModel=Trapezoidal non iterative  BusType=PV  Pref=3845e6  Qref=0  Qmin=-inf  Qmax=inf  PLF=0  QLF=0
  MTL Load : Subsystem
  NAN 1 : spsThreePhaseVIMeasurementLib/Three-Phase V-I Measurement  VoltageMeasurement=phase-to-ground  SetLabelV=on  LabelV=Vabc_NAN1  Vpu=off  VpuLL=off  CurrentMeasurement=no  SetLabelI=off  LabelI=Iabc  Ipu=off  Pbase=100e6  Vbase=500e3  OutputType=Complex  PhasorSimulation=off  PSBequivalent=0
  NAN-SAT 109 km : spsDistributedParametersLineLib/Distributed Parameters Line  Phases=3  Length=109  Frequency=60  Resistance=[0.01273 0.3864]/6  Inductance="[0.9337e-3  4.1264e-3]/6"  Capacitance=[12.74e-9 7.751e-9]*6  x1=[-0.00066 3.48177256927709e-08 0 0;-0.0006 3.55559771413437e-08 0 0;-0.00054 3.62760374950121e-08 0 0;-0.00048 3.69775383575939e-08 0 0;-0.00042 3.76601208282856e-08 -79004.1682206811 -247620.13099611;-0.00036 3.83234356852826e-08 -73383.4017976479 -249343.69646983;-0.0003 3.89671435644472e-08 -67725.0910702856 -250939.693101094;-0.00024 3.95909151329343e-08 -62032.1309349159 -252407.304348536;-0.00018 4.01944312576834e-08 -56307.434015138 -253745.779355121;-0.00012 4.07773831686934e-08 -50553.9291716762 -254954.433332306;-6e-05 4.13394726169948e-08 -44774.5600039209 -256032.647910382]  x2=[-0.00066 7.2071978897692e-09 0 0;-0.0006 6.57982450470479e-09 0 0;-0.00054 5.94908475984259e-09 0 0;-0.00048 5.31530135329082e-09 0 0;-0.00042 4.67879854035122e-09 -136734.260928183 -258979.315838023;-0.00036 4.03990196762412e-09 -130841.806753898 -262005.690696918;-0.0003 3.39893850640158e-09 -124882.411493599 -264898.018603144;-0.00024 2.756236085434e-09 -118859.124084018 -267654.8197883;-0.00018 2.11212352315573e-09 -112775.026150291 -270274.68382196;-0.00012 1.46693035945546e-09 -106633.230429344 -272756.270333275;-6e-05 8.20986687077529e-10 -100436.879177353 -275098.309696731]  x3=[-0.00066 2.00897624054229e-09 0 0;-0.0006 1.98364335424934e-09 0 0;-0.00054 1.95729559936285e-09 0 0;-0.00048 1.92994645588106e-09 0 0;-0.00042 1.90160991613113e-09 -4233.24689377981 3616.38239731893;-0.00036 1.8723004776104e-09 -4313.95722069102 3519.71148687609;-0.0003 1.84203313556918e-09 -4392.46044737536 3421.23982699977;-0.00024 1.81082337533895e-09 -4468.71641013149 3321.01779761072;-0.00018 1.77868716440973e-09 -4542.68609499982 3219.09667415106;-0.00012 1.74564094426084e-09 -4614.33165772275 3115.52860135083;-6e-05 1.71170162194912e-09 -4683.61644310654 3010.3665665498]  x4=[-0.00066 -1.68253194912286e-09 0 0;-0.0006 -1.65544140776799e-09 0 0;-0.00054 -1.62750391199985e-09 0 0;-0.00048 -1.59873375515753e-09 0 0;-0.00042 -1.56914565658486e-09 -1324.76102147867 -14462.5719103943;-0.00036 -1.53875475409981e-09 -997.314695297717 -14488.8362469249;-0.0003 -1.50757659624964e-09 -669.358124490388 -14507.6878271086;-0.00024 -1.47562713435601e-09 -341.059097698253 -14519.1170061288;-0.00018 -1.442922714354e-09 -12.5855787696892 -14523.1179366061;-0.00012 -1.40948006842917e-09 315.894379173529 -14519.6885715908;-6e-05 -1.37531630645714e-09 644.212719715304 -14508.8306656092]  x5=0.000616440308025359  V1=[4.327e-18 2.694e-07 2.694e-07;377 377 377;-0.06841 1.312 -0.2585]  V2=[4.095e-15 0.006804 0.006804;377 377 377;-0.7508 1.28 -0.2912]  I1=[2.296e-17 0.0001774 0.0001774;377 377 377;-2.081 -0.2552 -1.826]  I2=[2.168e-17 0.0001764 0.0001764;377 377 377;0.8233 2.744 1.174]  nHarmo=1  Measurements=None  Decoupling=off  VsMag0=0  VrMag0=0  VsAngle0=0  VrAngle0=0  IsMag0=0  IrMag0=0  IsAngle0=0  IrAngle0=0
      settings: LibrarySourceBlock=sps_lib/Power Grid Elements/Distributed Parameters Line
  North Network : Subsystem
  ORE-NAN 117 km3 : spsDistributedParametersLineLib/Distributed Parameters Line  Phases=3  Length=117  Frequency=60  Resistance=[0.01273 0.3864]/6  Inductance="[0.9337e-3  4.1264e-3]/6"  Capacitance=[12.74e-9 7.751e-9]*6  x1=[-0.00072 7.59022995949618e-10 0 0;-0.00066 2.36802768991538e-10 0 0;-0.0006 -2.85538610638769e-10 0 0;-0.00054 -8.07733903439727e-10 0 0;-0.00048 -1.32951594465048e-09 0 0;-0.00042 -1.85061778093732e-09 -95884.0918232771 -247693.861720886;-0.00036 -2.37077280697194e-09 -90257.3386372794 -249799.19107702;-0.0003 -2.88971490183168e-09 -84584.408129071 -251776.718551241;-0.00024 -3.40717856515184e-09 -78868.2026747236 -253625.432403953;-0.00018 -3.92289905296065e-09 -73111.646790571 -255344.386798987;-0.00012 -4.43661251312713e-09 -67317.6856369724 -256932.702287513;-6e-05 -4.94805612035272e-09 -61489.2835115141 -258389.566257978]  x2=[-0.00072 7.8308839392195e-09 0 0;-0.00066 7.2071978897692e-09 0 0;-0.0006 6.57982450470479e-09 0 0;-0.00054 5.94908475984259e-09 0 0;-0.00048 5.31530135329082e-09 0 0;-0.00042 4.67879854035122e-09 -136734.260928183 -258979.315838023;-0.00036 4.03990196762412e-09 -130841.806753898 -262005.690696918;-0.0003 3.39893850640158e-09 -124882.411493599 -264898.018603144;-0.00024 2.756236085434e-09 -118859.124084018 -267654.8197883;-0.00018 2.11212352315573e-09 -112775.026150291 -270274.68382196;-0.00012 1.46693035945546e-09 -106633.230429344 -272756.270333275;-6e-05 8.20986687077529e-10 -100436.879177353 -275098.309696731]  x3=[-0.00072 2.16877685746608e-10 0 0;-0.00066 2.16914240979666e-10 0 0;-0.0006 2.16839818878923e-10 0 0;-0.00054 2.16654457520103e-10 0 0;-0.00048 2.16358251737502e-10 0 0;-0.00042 2.15951353075471e-10 -4391.57203671345 585.606559686918;-0.00036 2.15433969710884e-10 -4403.69324163603 486.129825475721;-0.0003 2.14806366346631e-10 -4413.56143572529 386.404378263164;-0.00024 2.1406886407619e-10 -4421.1715702308 286.481239430755;-0.00018 2.1322184021935e-10 -4426.51975166712 186.411531502689;-0.00012 2.12265728129167e-10 -4429.6032438058 86.2464519906173;-6e-05 2.11201016970253e-10 -4430.4204690753 -13.9627527999441]  x4=[-0.00072 -9.68324126702992e-11 0 0;-0.00066 -1.05674218462107e-10 0 0;-0.0006 -1.14461959371114e-10 0 0;-0.00054 -1.23191139426693e-10 0 0;-0.00048 -1.31857292619031e-10 0 0;-0.00042 -1.40455985184022e-10 -1596.18035571344 -11376.948869749;-0.00036 -1.48982817871665e-10 -1338.45369527674 -11410.1411821858;-0.0003 -1.57433428196799e-10 -1080.04225719776 -11437.4958555586;-0.00024 -1.65803492671032e-10 -821.0782495431 -11458.9988947111;-0.00018 -1.74088729014719e-10 -561.694163084197 -11474.6392982911;-0.00012 -1.82284898347851e-10 -302.022703512545 -11484.4090643791;-6e-05 -1.90387807358752e-10 -42.1967235450385 -11488.3031945824]  x5=0.000661683633385019  V1=[2.771e-15 0.004375 0.004375;377 377 377;-0.7831 1.268 -0.3032]  V2=[4.095e-15 0.006804 0.006804;377 377 377;-0.7678 1.269 -0.3016]  I1=[9.029e-18 6.296e-05 6.296e-05;377 377 377;-1.689 -0.005215 -1.576]  I2=[6.955e-18 6.141e-05 6.141e-05;377 377 377;0.2743 2.461 0.89]  nHarmo=1  Measurements=None  Decoupling=off  VsMag0=0  VrMag0=0  VsAngle0=0  VrAngle0=0  IsMag0=0  IrMag0=0  IsAngle0=0  IrAngle0=0
      settings: LibrarySourceBlock=sps_lib/Power Grid Elements/Distributed Parameters Line
  OSI 1 : spsThreePhaseVIMeasurementLib/Three-Phase V-I Measurement  VoltageMeasurement=no  SetLabelV=on  LabelV=Vabc  Vpu=off  VpuLL=off  CurrentMeasurement=no  SetLabelI=off  LabelI=Iabc  Ipu=off  Pbase=100e6  Vbase=500e3  OutputType=Complex  PhasorSimulation=off  PSBequivalent=0
  OSI-MPO 187 km : spsDistributedParametersLineLib/Distributed Parameters Line  Phases=3  Length=187  Frequency=60  Resistance=[0.01273 0.3864]/6  Inductance="[0.9337e-3  4.1264e-3]/6"  Capacitance=[12.74e-9 7.751e-9]*6  x1=[-0.00108 1.17870798516311e-08 0 0;-0.00102 1.18266302577172e-08 0 0;-0.00096 1.18601299412325e-08 0 0;-0.0009 1.18875617631197e-08 0 0;-0.00084 1.19089116887521e-08 0 0;-0.00078 1.19241687951132e-08 0 0;-0.00072 1.19333252763853e-08 0 0;-0.00066 1.19363764479436e-08 -173678.926754002 -294540.651604074;-0.0006 1.19333207487522e-08 -166972.708064465 -298393.532624853;-0.00054 1.19241597421634e-08 -160181.063052182 -302093.750000664;-0.00048 1.19088981151173e-08 -153307.466448235 -305639.410631923;-0.00042 1.18875436757443e-08 -146355.434911658 -309028.700493136;-0.00036 1.18601073493704e-08 -139328.525230241 -312259.885560983;-0.0003 1.18266031729268e-08 -132230.332500822 -315331.312701478;-0.00024 1.17870482877696e-08 -125064.48828996 -318241.410515742;-0.00018 1.17414629309087e-08 -117834.658775963 -320988.690143961;-0.00012 1.1689870424655e-08 -110544.542873202 -323571.746027113;-6e-05 1.16322971646881e-08 -103197.870339678 -325989.256626079]  x2=[-0.00108 5.85669889392434e-09 0 0;-0.00102 5.75748418166442e-09 0 0;-0.00096 5.65532383411108e-09 0 0;-0.0009 5.55027011838585e-09 0 0;-0.00084 5.44237678191084e-09 0 0;-0.00078 5.33169902491065e-09 0 0;-0.00072 5.21829347217085e-09 0 0;-0.00066 5.1022181440677e-09 -171061.821363166 -279655.1295379;-0.0006 4.9835324268839e-09 -164692.945626598 -283452.624359401;-0.00054 4.86229704242542e-09 -158239.809935871 -287105.099580677;-0.00048 4.73857401695511e-09 -151705.715834446 -290610.686527916;-0.00042 4.61242664945895e-09 -145094.0062856 -293967.591678059;-0.00036 4.48391947926107e-09 -138408.06396211 -297174.097576403;-0.0003 4.3531182530043e-09 -131651.30951561 -300228.563715281;-0.00024 4.22008989101292e-09 -124827.199826525 -303129.427373376;-0.00018 4.084902453055e-09 -117939.226235468 -305875.204415239;-0.00012 3.94762510352178e-09 -110990.912757002 -308464.490050599;-6e-05 3.80832807604187e-09 -103985.814276693 -310895.959553081]  x3=[-0.00108 1.78220025588848e-10 0 0;-0.00102 1.75624891176319e-10 0 0;-0.00096 1.72939903824288e-10 0 0;-0.0009 1.701664372219e-10 0 0;-0.00084 1.67305910325914e-10 0 0;-0.00078 1.64359786634748e-10 0 0;-0.00072 1.61329573439719e-10 0 0;-0.00066 1.58216821053891e-10 -3246.80003615859 -6207.52765075389;-0.0006 1.55023122018902e-10 -3105.57039981553 -6279.37510080162;-0.00054 1.51750110290189e-10 -2962.75189627157 -6348.00990651825;-0.00048 1.48399460401033e-10 -2818.41759411212 -6413.39695306898;-0.00042 1.44972886605828e-10 -2672.64133743316 -6475.50278723257;-0.00036 1.41472142003045e-10 -2525.49770806123 -6534.29563451667;-0.0003 1.37899017638309e-10 -2377.06198739603 -6589.74541541426;-0.00024 1.34255341588068e-10 -2227.41011789501 -6641.82376079282;-0.00018 1.30542978024317e-10 -2076.61866421988 -6690.50402640857;-0.00012 1.26763826260852e-10 -1924.76477406463 -6735.76130653811;-6e-05 1.22919819781545e-10 -1771.9261386854 -6777.57244672067]  x4=[-0.00108 -3.80578575294307e-11 0 0;-0.00102 -3.53599990638576e-11 0 0;-0.00096 -3.26440497693858e-11 0 0;-0.0009 -2.99113991758592e-11 0 0;-0.00084 -2.71634453578152e-11 0 0;-0.00078 -2.44015942192034e-11 0 0;-0.00072 -2.16272587740994e-11 0 0;-0.00066 -1.88418584237807e-11 -5891.26575595252 -5505.05705820958;-0.0006 -1.6046818230535e-11 -5765.24750678464 -5636.89555793102;-0.00054 -1.32435681885714e-11 -5636.27965046275 -5765.85011772717;-0.00048 -1.04335424924095e-11 -5504.42816932521 -5891.85476206243;-0.00042 -7.61817880311881e-12 -5369.76052102611 -6014.84502463245;-0.00036 -4.79891751278469e-12 -5232.34560402269 -6134.75798134632;-0.0003 -1.97720100757722e-12 -5092.25372232562 -6251.53228251964;-0.00024 8.45527070200198e-13 -4949.55654953017 -6365.10818426219;-0.00018 3.66782256070496e-12 -4804.3270921467 -6475.42757904399;-0.00012 6.48824152541409e-12 -4656.63965224912 -6582.43402542421;-6e-05 9.3053409858699e-12 -4506.56978946065 -6686.07277692762]  x5=0.00105756273028204  V1=[3.05e-13 0.3186 0.3186;377 377 377;-0.6471 -1.909 2.804]  V2=[3.793e-13 0.4417 0.4417;377 377 377;-0.6023 -1.906 2.806]  I1=[5.824e-16 0.002377 0.002377;377 377 377;-1.191 -2.924 1.788]  I2=[4.03e-16 0.002279 0.002279;377 377 377;-0.283 -1.078 -2.649]  nHarmo=1  Measurements=None  Decoupling=off  VsMag0=0  VrMag0=0  VsAngle0=0  VrAngle0=0  IsMag0=0  IrMag0=0  IsAngle0=0  IrAngle0=0
      settings: LibrarySourceBlock=sps_lib/Power Grid Elements/Distributed Parameters Line
  PSS : Constant
  PSS_Equation : Subsystem
  Regulators 10 : Subsystem
  South Network : Subsystem
  Stair Generator : eeStairGenerator/Stair Generator  LabelModeActiveChoice=Discrete  TimeInput=[0.1 0.15 0.2]  AmplitudeInput=[0 1 0]  SampleTime=-1  RepeatPattern=off  OutDataTypeStr=double
      settings: LibrarySourceBlock=ee_sl_lib/General Control/Stair Generator
  Three-Phase Fault : spsThreePhaseFaultLib/Three-Phase Fault  InitialStates=0  FaultA=on  FaultB=on  FaultC=on  GroundFault=on  SwitchTimes="[0.2  0.4]"  External=on  SwitchStatus=NaN  FaultResistance=0.001  GroundResistance=0.01  SnubberResistance=1e6  SnubberCapacitance=inf  Measurements=None
  powergui : sps_lib/powergui  Priority=1  SimulationMode=Discrete  SampleTime=6e-5  frequency=60  Iterations=50  frequencyindice=0  Pbase=100e6  ErrMax=1e-4  UnitsV=kV  UnitsW=MW  buscounter=0  FunctionMessages=off  echomessages=off  EnableUseOfTLC=off  CurrentSourceSwitches=off  DisableSnubberDevices=off  DisableRonSwitches=off  DisableVfSwitches=off  DisplayEquations=off  AutomaticDiscreteSolvers=off  SolverType=Tustin/Backward Euler (TBE)  Interpol=off  ExternalGateDelay=off  methode=off  Ts=100  x0status=blocks  SPID=on  SwTol=0  HookPort=off  NonlinearTolerance=1e-4  nMaxIteration=100  ContinueOnMaxIteration=off  RestoreLinks=warning  ResistiveCurrentMeasurement=off  Frange=[0:2:500]  Ylog=off  Xlog=on  ShowGrid=off  save=off  variable=ZData  structure=0  ZoomFFT=off  StartTime=0.0  cycles=1  DisplayStyle=1  fundamental=60  FreqAxis=off  MaxFrequency=1000  frequencyindicesteady=1  RmsSteady=1  display=off
  wires:
  PSS/1 -> PSS_Equation/1(In1)
  Regulators 10/1(Pm) -> MPP7 4700 MVA 17KV/1
  MPP7 4700 MVA 17KV/1 -> Regulators 10/1(m)
  Regulators 10/2(Vf) -> MPP7 4700 MVA 17KV/2
  Stair Generator/1 -> Three-Phase Fault/1
  connections:
  South Network/LConn3 -- CON-OSI 144 km/RConn3
  South Network/LConn2 -- CON-OSI 144 km/RConn2
  South Network/LConn1 -- CON-OSI 144 km/RConn1
  OSI 1/LConn1 -- CON-OSI 144 km/LConn1
  CON-OSI 144 km/LConn2 -- OSI 1/LConn2
  CON-OSI 144 km/LConn3 -- OSI 1/LConn3
  Cs OSIS/LConn1 -- OSI 1/RConn1
  Cs OSIS/LConn2 -- OSI 1/RConn2
  Cs OSIS/LConn3 -- OSI 1/RConn3
  150 MW/LConn1 -- MPP7 4700 MVA 17KV/RConn1 -- "4700 MVA 17KV :650KV Transformer "/LConn1 -- Load Flow Bus1/LConn1
  150 MW/LConn2 -- MPP7 4700 MVA 17KV/RConn2 -- "4700 MVA 17KV :650KV Transformer "/LConn2
  "4700 MVA 17KV :650KV Transformer "/LConn3 -- MPP7 4700 MVA 17KV/RConn3 -- 150 MW/LConn3
  North Network/RConn1 -- ATL-MPO 350 km/RConn1
  Cs OSIS/RConn1 -- Load Flow Bus3/LConn1 -- OSI-MPO 187 km/LConn1
  Cs OSIS/RConn2 -- OSI-MPO 187 km/LConn2
  Cs OSIS/RConn3 -- OSI-MPO 187 km/LConn3
  MPP10-MPO 234 km/LConn1 -- 330 MVar/LConn1 -- "4700 MVA 17KV :650KV Transformer "/RConn1
  MPP10-MPO 234 km/LConn2 -- 330 MVar/LConn2 -- "4700 MVA 17KV :650KV Transformer "/RConn2
  MPP10-MPO 234 km/LConn3 -- "4700 MVA 17KV :650KV Transformer "/RConn3 -- 330 MVar/LConn3
  MPP10-MPO 234 km/RConn1 -- " 41.4 MW Wind Generation"/LConn1 -- Li-ion BESS/LConn1 -- OSI-MPO 187 km/RConn1 -- 400 kV Solar Farm/LConn1 -- Cs MPOD/RConn1 -- Load Flow Bus2/LConn1
  MPP10-MPO 234 km/RConn2 -- Li-ion BESS/LConn2 -- OSI-MPO 187 km/RConn2 -- " 41.4 MW Wind Generation"/LConn2 -- 400 kV Solar Farm/LConn2 -- Cs MPOD/RConn2
  MPP10-MPO 234 km/RConn3 -- Li-ion BESS/LConn3 -- OSI-MPO 187 km/RConn3 -- " 41.4 MW Wind Generation"/LConn3 -- 400 kV Solar Farm/LConn3 -- Cs MPOD/RConn3
  MPO 3/RConn1 -- ATL-MPO 350 km/LConn1 -- Cs MPOD/LConn1
  MPO 3/RConn2 -- ATL-MPO 350 km/LConn2 -- Cs MPOD/LConn2
  MPO 3/RConn3 -- ATL-MPO 350 km/LConn3 -- Cs MPOD/LConn3
  NAN 1/LConn2 -- Home Network Load （with circuit breaker)/LConn2 -- MTL Load/LConn2 -- Three-Phase Fault/LConn2 -- NAN-SAT 109 km/RConn2 -- MPO-NAN 277 km/RConn2
  MTL Load/LConn1 -- Home Network Load （with circuit breaker)/LConn1 -- Load Flow Bus5/LConn1 -- Three-Phase Fault/LConn1 -- Load Flow Bus4/LConn1 -- NAN-SAT 109 km/RConn1 -- MPO-NAN 277 km/RConn1 -- NAN 1/LConn1
  ATL-MPO 350 km/RConn2 -- North Network/RConn2
  North Network/RConn3 -- ATL-MPO 350 km/RConn3
  North Network/LConn1 -- ORE-NAN 117 km3/LConn1
  North Network/LConn2 -- ORE-NAN 117 km3/LConn2
  North Network/LConn3 -- ORE-NAN 117 km3/LConn3
  NAN 1/RConn3 -- ORE-NAN 117 km3/RConn3
  ORE-NAN 117 km3/RConn2 -- NAN 1/RConn2
  ORE-NAN 117 km3/RConn1 -- NAN 1/RConn1
  South Network/LConn4 -- NAN-SAT 109 km/LConn1
  South Network/LConn5 -- NAN-SAT 109 km/LConn2
  South Network/LConn6 -- NAN-SAT 109 km/LConn3
  MPO-NAN 277 km/LConn3 -- 660 MVar/LConn3 -- MPO 3/LConn3
  MPO 3/LConn2 -- 660 MVar/LConn2 -- MPO-NAN 277 km/LConn2
  MPO-NAN 277 km/LConn1 -- 660 MVar/LConn1 -- MPO 3/LConn1
  MPO-NAN 277 km/RConn3 -- NAN-SAT 109 km/RConn3 -- Home Network Load （with circuit breaker)/LConn3 -- MTL Load/LConn3 -- Three-Phase Fault/LConn3 -- NAN 1/LConn3
